simulink model "pid_controller"  (R2018a)
settings: Solver=VariableStepAuto  StartTime=0.0  StopTime=50  MaxStep=0.01  RelTol=1e-4  EnableMultiTasking=on
libraries: simulink x2
settings Model: Creator=Rafael  LastModifiedBy=Rafael
settings DataIOCC: LimitDataPoints=on  SaveOutput=off  SaveTime=off
settings OptimizationCC: ExpressionDepthLimit=2147483647  LifeSpan=1
settings DebuggingCC: UnderspecifiedInitializationDetection=Classic  MergeDetectMultiDrivingBlocksExec=none  FcnCallInpInsideContextMsg=warning  AllowSymbolicDim=off  StateNameClashWarn=warning  SFUnexpectedBacktrackingDiag=warning  SFNoUnconditionalDefaultTransitionDiag=warning  SFExecutionAtInitializationDiag=none
settings CodeAppCC: StateflowObjectComments=on
settings GRTTargetCC: TargetLangStandard=C89/C90 (ANSI)  GeneratePreprocessorConditionals=Disable all  CombineOutputUpdateFcns=off  GRTInterface=on

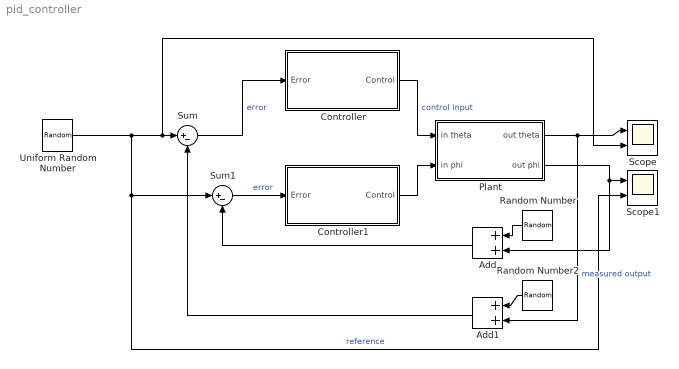
== system pid_controller ==
  Add : Sum
  Add1 : Sum
  Controller : Subsystem
  Controller1 : Subsystem
  Plant : Subsystem
  Random Number : RandomNumber  Variance=0.01  SampleTime=0.1
  Random Number2 : RandomNumber  Variance=0.01  SampleTime=0.1
  Scope : Scope  NumInputPorts=2
  Scope1 : Scope  NumInputPorts=2
  Sum : Sum  Inputs=|+-
  Sum1 : Sum  Inputs=|+-
  Uniform Random Number : UniformRandomNumber  Minimum=-45  Maximum=45  SampleTime=0.1
  wires:
  Plant/1(out theta) -> Add1/2, Scope/1  "measured output"
  Sum/1 -> Controller/1(Error)  "error"
  Controller/1(Control) -> Plant/1(in theta)  "control input"
  Plant/2(out phi) -> Add/2, Scope1/1
  Uniform Random Number/1 -> Scope1/2, Sum1/1, Scope/2, Sum/1  "reference"
  Sum1/1 -> Controller1/1(Error)  "error"
  Controller1/1(Control) -> Plant/2(in phi)
  Random Number/1 -> Add/1
  Add/1 -> Sum1/2
  Random Number2/1 -> Add1/1
  Add1/1 -> Sum/2

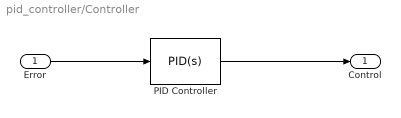
== system pid_controller/Controller ==
  Error : Inport
  PID Controller : simulink/Continuous/PID Controller  Controller=PID  TimeDomain=Continuous-time  SampleTime=-1  IntegratorMethod=Forward Euler  FilterMethod=Forward Euler  Form=Parallel  UseFilter=on  ControllerParametersSource=internal  P=-1.08e+05  I=-1.12e+07  D=-260  N=1e+5  InitialConditionSource=internal  InitialConditionForIntegrator=0  InitialConditionForFilter=0  ExternalReset=none  LimitOutput=off  UpperSaturationLimit=inf  LowerSaturationLimit=-inf  LinearizeAsGain=on  AntiWindupMode=none  Kb=1  TrackingMode=off  Kt=1  PParamMin=[]  PParamMax=[]  IParamMin=[]  IParamMax=[]  DParamMin=[]  DParamMax=[]  NParamMin=[]  NParamMax=[]  KbParamMin=[]  KbParamMax=[]  KtParamMin=[]  KtParamMax=[]  POutMin=[]  POutMax=[]  IOutMin=[]  IOutMax=[]  DOutMin=[]  DOutMax=[]  NOutMin=[]  NOutMax=[]  KbOutMin=[]  KbOutMax=[]  KtOutMin=[]  KtOutMax=[]  IntegratorOutMin=[]  IntegratorOutMax=[]  FilterOutMin=[]  FilterOutMax=[]  SumOutMin=[]  SumOutMax=[]  SumI1OutMin=[]  SumI1OutMax=[]  SumI2OutMin=[]  SumI2OutMax=[]  SumI3OutMin=[]  SumI3OutMax=[]  SumDOutMin=[]  SumDOutMax=[]  SaturationOutMin=[]  SaturationOutMax=[]  IntegratorContinuousStateAttributes=''  IntegratorStateMustResolveToSignalObject=off  IntegratorRTWStateStorageClass=Auto  FilterContinuousStateAttributes=''  FilterStateMustResolveToSignalObject=off  FilterRTWStateStorageClass=Auto  DifferentiatorICPrevScaledInput=0  DifferentiatorOutMin=[]  DifferentiatorOutMax=[]  FilterDiffOutCoefMin=[]  FilterDiffOutCoefMax=[]  SumDenOutMin=[]  SumDenOutMax=[]  SumNumOutMin=[]  SumNumOutMax=[]  ReciprocalOutMin=[]  ReciprocalOutMax=[]  DivideOutMin=[]  DivideOutMax=[]  TunerSelectOption=Transfer Function Based (PID Tuner App)
  Control : Outport
  wires:
  Error/1 -> PID Controller/1
  PID Controller/1 -> Control/1

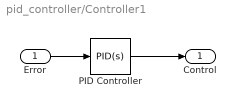
== system pid_controller/Controller1 ==
  Error : Inport
  PID Controller : simulink/Continuous/PID Controller  Controller=PID  TimeDomain=Continuous-time  SampleTime=-1  IntegratorMethod=Forward Euler  FilterMethod=Forward Euler  Form=Parallel  UseFilter=on  ControllerParametersSource=internal  P=4.17e+04  I=3.56e+06  D=122  N=1e+5  InitialConditionSource=internal  InitialConditionForIntegrator=0  InitialConditionForFilter=0  ExternalReset=none  LimitOutput=off  UpperSaturationLimit=inf  LowerSaturationLimit=-inf  LinearizeAsGain=on  AntiWindupMode=none  Kb=1  TrackingMode=off  Kt=1  PParamMin=[]  PParamMax=[]  IParamMin=[]  IParamMax=[]  DParamMin=[]  DParamMax=[]  NParamMin=[]  NParamMax=[]  KbParamMin=[]  KbParamMax=[]  KtParamMin=[]  KtParamMax=[]  POutMin=[]  POutMax=[]  IOutMin=[]  IOutMax=[]  DOutMin=[]  DOutMax=[]  NOutMin=[]  NOutMax=[]  KbOutMin=[]  KbOutMax=[]  KtOutMin=[]  KtOutMax=[]  IntegratorOutMin=[]  IntegratorOutMax=[]  FilterOutMin=[]  FilterOutMax=[]  SumOutMin=[]  SumOutMax=[]  SumI1OutMin=[]  SumI1OutMax=[]  SumI2OutMin=[]  SumI2OutMax=[]  SumI3OutMin=[]  SumI3OutMax=[]  SumDOutMin=[]  SumDOutMax=[]  SaturationOutMin=[]  SaturationOutMax=[]  IntegratorContinuousStateAttributes=''  IntegratorStateMustResolveToSignalObject=off  IntegratorRTWStateStorageClass=Auto  FilterContinuousStateAttributes=''  FilterStateMustResolveToSignalObject=off  FilterRTWStateStorageClass=Auto  DifferentiatorICPrevScaledInput=0  DifferentiatorOutMin=[]  DifferentiatorOutMax=[]  FilterDiffOutCoefMin=[]  FilterDiffOutCoefMax=[]  SumDenOutMin=[]  SumDenOutMax=[]  SumNumOutMin=[]  SumNumOutMax=[]  ReciprocalOutMin=[]  ReciprocalOutMax=[]  DivideOutMin=[]  DivideOutMax=[]  TunerSelectOption=Transfer Function Based (PID Tuner App)
  Control : Outport
  wires:
  Error/1 -> PID Controller/1
  PID Controller/1 -> Control/1

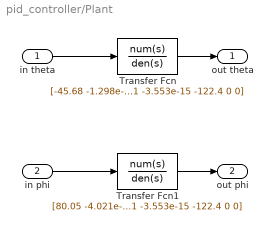
== system pid_controller/Plant ==
  in theta : Inport
  in phi : Inport  Port=2
  Transfer Fcn : TransferFcn  Numerator=[-45.68 -1.298e-11 7.179e-13]  Denominator=[1 -3.553e-15 -122.4 0 0]
  Transfer Fcn1 : TransferFcn  Numerator=[80.05 -4.021e-12 61140]  Denominator=[1 -3.553e-15 -122.4 0 0]
  out theta : Outport
  out phi : Outport  Port=2
  wires:
  in theta/1 -> Transfer Fcn/1
  in phi/1 -> Transfer Fcn1/1
  Transfer Fcn1/1 -> out phi/1
  Transfer Fcn/1 -> out theta/1
